simulink model "test_controlador_hoist"  (R2023b)
settings: Solver=FixedStepAuto  StartTime=0.0  StopTime=10.0  FixedStep=0.001  RelTol=1e-3
settings Model: Creator=Ferran  LastModifiedBy=Ferran

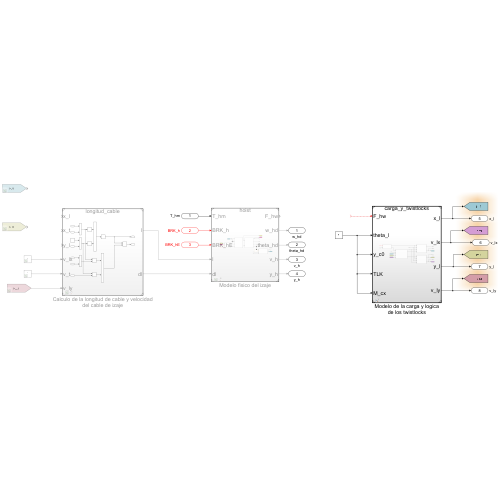
[thumbnail: Simulink's stored preview of the top-level diagram]
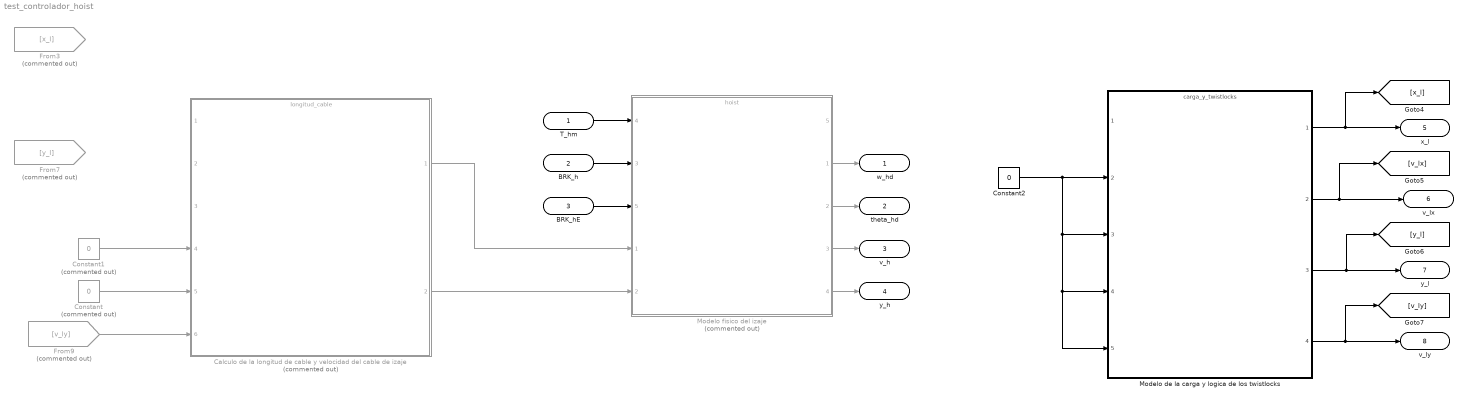
== system test_controlador_hoist ==
  T_hm : Inport
  BRK_h : Inport  Port=2
  BRK_hE : Inport  Port=3
  Calculo de la longitud de cable y velocidad del cable de izaje : ModelReference  Commented=on  ModelNameDialog=longitud_cable.slx  SimulationMode=Normal  ModelReferenceVersion=1.4
  Constant : Constant  Commented=on  Value=0
  Constant1 : Constant  Commented=on  Value=0
  Constant2 : Constant  Value=0
  From3 : From  Commented=on  GotoTag=x_l
  From7 : From  Commented=on  GotoTag=y_l
  From9 : From  Commented=on  GotoTag=v_ly
  Modelo de la carga y logica de los twistlocks : ModelReference  ModelNameDialog=carga_y_twistlocks.slx  SimulationMode=Normal  ModelReferenceVersion=1.14
  Modelo fisico del izaje : ModelReference  Commented=on  ModelNameDialog=hoist.slx  SimulationMode=Normal  ModelReferenceVersion=1.22
      settings: PortSchema="{\"entries\":[{\"content\":{\"sides\":[{\"content\":{\"connectorIds\":[\"In4\",\"In3\",\"In5\",\"In1\",\"In2\"]},\"type\":\"ConnectorPlacement.EquallySpacedRectSide\",\"uuid\":\"17f6338c-3c51-40de-9973-080572c91603\"},{\"content\":{\"connectorIds\":[\"Out5\",\"Out1\",\"Out2\",\"Out3\",\"Out4\"],\"side\":\"RIGHT\"},\"type\":\"ConnectorPlacement.EquallySpacedRectSide\",\"uuid\":\"7e968b16-4cea-43bb-a5ca-e4df3289f40a\"},{\"content\":{\"side\":\"TOP\"},\"type\":\"ConnectorPlacement.EquallySpacedRectSide\",\"uuid\":\"93c8c357-b571-41b6-8c5b-1c91e217cb64\"}]},\"type\":\"ConnectorPlacement.EquallySpacedConnector\",\"uuid\":\"e66d9c43-4482-4d93-9c83-496ca9c2d477\"}],\"packageUris\":[\"http://schema.mathworks.com/mf0/Connector/R2020b\"],\"version\":\"1.0\"}"
  w_hd : Outport
  theta_hd : Outport  Port=2
  v_h : Outport  Port=3
  y_h : Outport  Port=4
  x_l : Outport  Port=5
  v_lx : Outport  Port=6
  y_l : Outport  Port=7
  v_ly : Outport  Port=8
  wires:
  From9/1 -> Calculo de la longitud de cable y velocidad del cable de izaje/6
  Modelo fisico del izaje/1 -> w_hd/1
  Modelo fisico del izaje/4 -> y_h/1
  Modelo fisico del izaje/2 -> theta_hd/1
  ? -> Modelo de la carga y logica de los twistlocks/1
  Modelo fisico del izaje/3 -> v_h/1
  Constant/1 -> Calculo de la longitud de cable y velocidad del cable de izaje/5
  Modelo de la carga y logica de los twistlocks/2 -> v_lx/1, [v_lx]
  Modelo de la carga y logica de los twistlocks/4 -> v_ly/1, [v_ly]
  T_hm/1 -> Modelo fisico del izaje/4
  Modelo de la carga y logica de los twistlocks/3 -> y_l/1, [y_l]
  Constant2/1 -> Modelo de la carga y logica de los twistlocks/3, Modelo de la carga y logica de los twistlocks/4, Modelo de la carga y logica de los twistlocks/5, Modelo de la carga y logica de los twistlocks/2
  Calculo de la longitud de cable y velocidad del cable de izaje/2 -> Modelo fisico del izaje/2
  BRK_hE/1 -> Modelo fisico del izaje/5
  BRK_h/1 -> Modelo fisico del izaje/3
  Modelo de la carga y logica de los twistlocks/1 -> x_l/1, [x_l]
  Constant1/1 -> Calculo de la longitud de cable y velocidad del cable de izaje/4
  Calculo de la longitud de cable y velocidad del cable de izaje/1 -> Modelo fisico del izaje/1
